simulink model "buegeleisen"  (R2020b)
settings: Solver=ode4  StartTime=0.0  StopTime=t  FixedStep=0.1  RelTol=1e-3
values from neighbouring files (symbols this model uses):
  A = 0.05    [init_buegeleisen.m]    (also in init_iron.m)
  alpha = 15    [init_buegeleisen.m]    (also in init_iron.m)
  cp = 449    [init_buegeleisen.m]    (also in init_iron.m)
  m = 0.5    [init_buegeleisen.m]    (also in init_iron.m)
  PB = 1000    [init_buegeleisen.m]    (also in init_iron.m)
  Tdiff = 10    [init_buegeleisen.m]    (also in init_iron.m)
  Tsoll = 100    [init_buegeleisen.m]
  Tumg = 20    [init_buegeleisen.m]
settings Model: Creator=root  LastModifiedBy=root

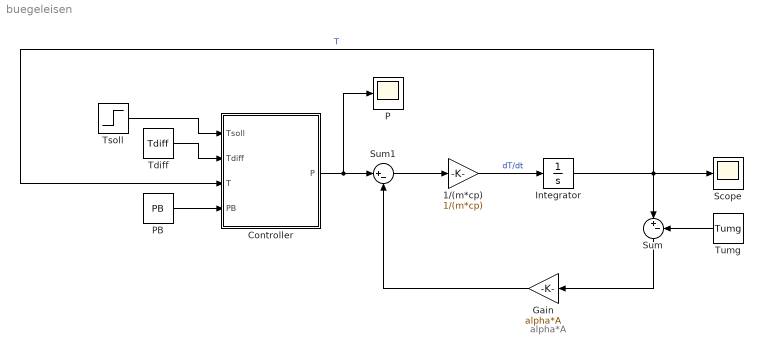
== system buegeleisen ==
  note: alpha*A
  1/(m*cp) : Gain  Gain=1/(m*cp)
  Controller : Stateflow chart  TreatAsAtomicUnit=on
  Gain : Gain  Gain=alpha*A
  Integrator : Integrator  InitialCondition=Tumg
  P : Scope
  PB : Constant  Value=PB
  Scope : Scope
  Sum : Sum  Inputs=|+-
  Sum1 : Sum  Inputs=|+-
  Tdiff : Constant  Value=Tdiff
  Tsoll : Step  Time=0  After=Tsoll  SampleTime=0
  Tumg : Constant  Value=Tumg
  wires:
  1/(m*cp)/1 -> Integrator/1  "dT/dt"
  Integrator/1 -> Controller/3(T), Sum/1, Scope/1  "T"
  Tumg/1 -> Sum/2
  Sum/1 -> Gain/1
  Gain/1 -> Sum1/2
  Sum1/1 -> 1/(m*cp)/1
  Tsoll/1 -> Controller/1(Tsoll)
  Tdiff/1 -> Controller/2(Tdiff)
  Controller/1(P) -> P/1, Sum1/1
  PB/1 -> Controller/4(PB)

== stateflow chart buegeleisen/Controller ==
  state ZU
    P=PB;
  state AUF
    P=0;
  ZU -> AUF : [T > Tsoll ]
  AUF -> ZU : [T<Tsoll-Tdiff]
  (default) -> AUF
  data: Tsoll input; Tdiff input; T input; P output; PB input
